simulink model "Inter_story_damped_structure_MBW_reference"  (R2023a)
settings: Solver=ode4  StartTime=0.0  StopTime=tend  FixedStep=dt  RelTol=1e-3
values from neighbouring files (symbols this model uses):
  A0 = 0.4    [Base_isolated_structure_main.m]    (also in Inter_story_damped_structure_MBW_main.m = [zeros(Ns) eye(Ns);-M\K -M\C]; Inter_story_damped_structure_MFD_main.m = [zeros(Ns) eye(Ns);-M\K -M\C])
  alpha = 0.52    [BLWN_training_data_prep.m]    (also in Base_isolated_structure_main.m; Inter_story_damped_structure_MBW_main.m = 4; Inter_story_damped_structure_MFD_main.m)
  B1 = [zeros(Ns,1+Ns);-ones(Ns,1) -M\Re]    [Inter_story_damped_structure_MBW_main.m]    (also in Inter_story_damped_structure_MFD_main.m)
  C0 = eye(2*Ns)    [Inter_story_damped_structure_MBW_main.m]    (also in Inter_story_damped_structure_MFD_main.m)
  CoeB = [A0,gamma,beta,n]    [Base_isolated_structure_main.m]    (also in Inter_story_damped_structure_MBW_main.m = [A,gamma,beta,n])
  CoeZ = [a,b,k1]    [Base_isolated_structure_main.m]    (also in Inter_story_damped_structure_MBW_main.m)
  D1 = zeros(2*Ns,1+Ns)    [Inter_story_damped_structure_MBW_main.m]    (also in Inter_story_damped_structure_MFD_main.m)
  dt = 0.002    [BLWN_training_data_prep.m]    (also in Base_isolated_structure_main.m; Inter_story_damped_structure_MBW_main.m; Inter_story_damped_structure_MFD_main.m)
  Ns = 5    [Inter_story_damped_structure_MBW_main.m]    (also in Inter_story_damped_structure_MFD_main.m)
settings Model: Creator=hongwei  LastModifiedBy=li292
settings DataIOCC: SaveTime=off  ReturnWorkspaceOutputs=off
settings OptimizationCC: ReuseModelBlockBuffer=off

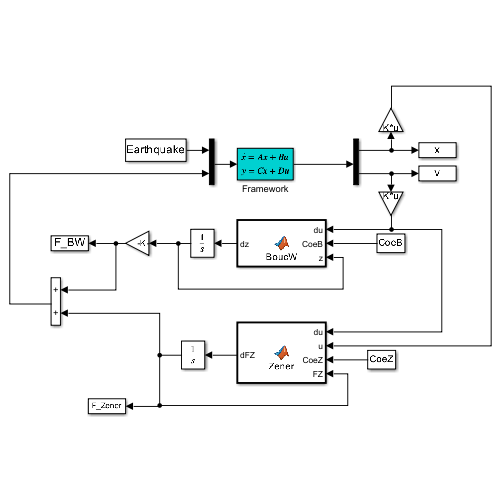
[thumbnail: Simulink's stored preview of the top-level diagram]
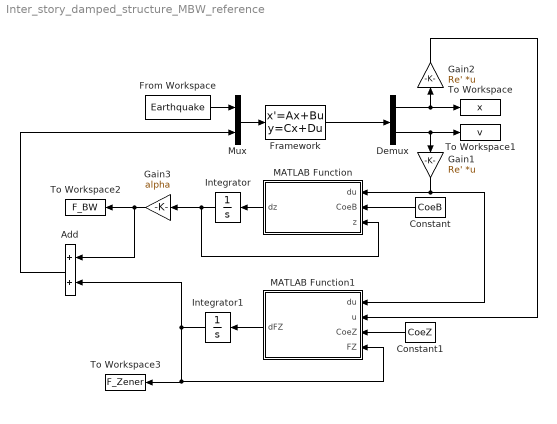
== system Inter_story_damped_structure_MBW_reference ==
  Add : Sum
  Constant : Constant  Value=CoeB
  Constant1 : Constant  Value=CoeZ
  Demux : Demux  Outputs=2
  Framework : StateSpace  A=A0  B=B1  C=C0  D=D1  InitialCondition=zeros(2*Ns,1)
  From Workspace : FromWorkspace  VariableName=Earthquake  SampleTime=dt
  Gain1 : Gain  Gain=Re'  Multiplication=Matrix(K*u)
  Gain2 : Gain  Gain=Re'  Multiplication=Matrix(K*u)
  Gain3 : Gain  Gain=alpha
  Integrator : Integrator  InitialCondition=zeros(Ns,1)
  Integrator1 : Integrator  InitialCondition=zeros(Ns,1)
  MATLAB Function : MATLAB Function  TreatAsAtomicUnit=on
  MATLAB Function1 : MATLAB Function  TreatAsAtomicUnit=on
  Mux : Mux  Inputs=2
  To Workspace : ToWorkspace  VariableName=x  SampleTime=-1
  To Workspace1 : ToWorkspace  VariableName=v  SampleTime=-1
  To Workspace2 : ToWorkspace  VariableName=F_BW  SampleTime=-1
  To Workspace3 : ToWorkspace  VariableName=F_Zener  SampleTime=-1
  wires:
  Framework/1 -> Demux/1
  Demux/1 -> Gain2/1, To Workspace/1
  Demux/2 -> To Workspace1/1, Gain1/1
  Mux/1 -> Framework/1
  Constant/1 -> MATLAB Function/2(CoeB)
  MATLAB Function/1(dz) -> Integrator/1
  From Workspace/1 -> Mux/1
  Add/1 -> Mux/2
  Gain2/1 -> MATLAB Function1/2(u)
  Constant1/1 -> MATLAB Function1/3(CoeZ)
  MATLAB Function1/1(dFZ) -> Integrator1/1
  Integrator1/1 -> To Workspace3/1, MATLAB Function1/4(FZ), Add/2
  Integrator/1 -> Gain3/1, MATLAB Function/3(z)
  Gain3/1 -> Add/1, To Workspace2/1
  Gain1/1 -> MATLAB Function/1(du), MATLAB Function1/1(du)

== matlab function Inter_story_damped_structure_MBW_reference/MATLAB Function1 ==
  data: du input; u input; CoeZ input; dFZ output; FZ input
function dFZ = Zener(du,u,CoeZ,FZ)
% CoeZ=[a,b,k1];
% Zener=@(du,u,f)b*u+k1*du-a*f;
a=CoeZ(1);
b=CoeZ(2);
k1=CoeZ(3);
dFZ=b*u+k1*du-a*FZ;

== matlab function Inter_story_damped_structure_MBW_reference/MATLAB Function ==
  data: du input; dz output; CoeB input; z input
function dz = BoucW(du,CoeB,z)
% coe=[A,gamma,beta,n];
% BoucW=@(du,z)-gamma*abs(du)*abs(z)^(n-1)*z-beta*du*abs(z)^n+A*du;
A=CoeB(1);
gamma=CoeB(2);
beta=CoeB(3);
n=CoeB(4);
dz=-gamma*abs(du).*abs(z).^(n-1).*z-beta*du.*abs(z).^n+A*du;
